simulink library "Kitchen_Lib"  (R2023a)
settings: Solver=VariableStepAuto  StartTime=0.0  StopTime=10.0  RelTol=1e-3  EnableMultiTasking=on
undefined symbols (not defined in the file): Kitc_BusTyp_P, Kitc_BusTypSkyr_C, Kitc_ColrLedColrls_C, Kitc_ColrLedGrn_C, Kitc_ColrLedRed_C, Kitc_ColrLedYlw_C, Kitc_StDgnWtrTank_C, Kitc_StElecPlugScktOffByClmp50_P, Kitc_StsDlyBlink_C, Kitc_StsErrBlink_C, Kitc_StsFctAcvn_P, Kitc_StsInfoBlink_C, Kitc_StsKitchnOffAutoIgOff_P, Kitc_StsKitchnOffBySwt_P, Kitc_StsKitchnOffDoorLockd_P, Kitc_StsKitchnOffIgOff_P, Kitc_StsKitchnOffUv_P, Kitc_StsKitchnOnBySwt_P, Kitc_StsKitchnOnNVM_P, Kitc_StsLedOff_C, Kitc_StsLedOn_C, Kitc_StsLrgCnsAcv_P, Kitc_StTrfrAnSwtInstd_P, Kitc_StTrfrSwtInstd_P, Kitc_TiKitcRefgtrOffDly_P, Kitc_ULowrThdBat_C, Kitc_UUpprThdBat_C, Kitc_ValFalse_C, Kitc_ValPwmFreq2_C, Kitc_ValPwmFreq_C, Kitc_ValTrue_C
libraries: MAN_Library x50, E2E_Lib x3
(part 8 of 13)

== system Kitchen_Lib/Kitchen/100ms/Kitchn/Subsystem1/Subsystem19/KSW_Battery/BatteryVoltageUnder23V/TurnOffDelay ==
  TurnOffDelayEnable : Inport
  TurnOffDelayThreshold : Inport  Port=2
  Constant1 : Constant  Value=uint32(100)  OutDataTypeStr=uint32
  Constant10 : Constant  Value=uint32(CycleTime)  OutDataTypeStr=uint32
  Constant11 : Constant  Value=uint32(1)  OutDataTypeStr=uint32
  Constant12 : Constant  Value=uint32(10)  OutDataTypeStr=uint32
  Constant13 : Constant  Value=uint32(100)  OutDataTypeStr=uint32
  Constant14 : Constant  Value=uint32(1000)  OutDataTypeStr=uint32
  Multiport Switch2 : MultiPortSwitch  Inputs=4  SaturateOnIntegerOverflow=off  InputSameDT=off
  Terminator : Terminator
  TurnOffDelayOriginal : Subsystem  AncestorBlock=MAN_Library/BasicLibrary/TurnOffDelayOriginal
  TurnOffDelayFlag : Outport
  TurnOffDelayExpiredTime : Outport  Port=2
  wires:
  TurnOffDelayOriginal/2(TurnOffDelayExpiredTime) -> TurnOffDelayExpiredTime/1
  TurnOffDelayOriginal/1(TurnOffDelayFlag) -> TurnOffDelayFlag/1
  TurnOffDelayThreshold/1 -> TurnOffDelayOriginal/2(TurnOffDelayThreshold)
  TurnOffDelayEnable/1 -> TurnOffDelayOriginal/1(TurnOffDelayEnable)
  Constant11/1 -> Multiport Switch2/2
  Constant12/1 -> Multiport Switch2/3
  Constant14/1 -> Multiport Switch2/5
  Constant13/1 -> Multiport Switch2/4
  Constant10/1 -> Multiport Switch2/1
  Multiport Switch2/1 -> Terminator/1
  Constant1/1 -> TurnOffDelayOriginal/3(CycleTime)

== system Kitchen_Lib/Kitchen/100ms/Kitchn/Subsystem1/Subsystem19/KitchenEnable/001_HostessSideButton/001_HostessSideTopButton ==
  note: Parameter G_78_PARA_Enable_KuecheBeif_S is deleted
  note: Parameter
      | G_78_PARA_Enable_KuecheBeif_S
      | is deleted
  Kitc_StKitcHostsSideSwtUpprPart : Inport
  SwtLock : Inport  Port=2
  "GW_ModeExbn " : Inport  Port=3
  "GW_StUvTopPrio " : Inport  Port=4
  Constant1 : Constant  Value=Kitc_ValFalse_C
  Logical Operator10 : Logic  Operator=NOT  Inputs=4  AllPortsSameDT=off  OutDataTypeStr=boolean
  Logical Operator11 : Logic  Operator=OR  Inputs=3  AllPortsSameDT=off  OutDataTypeStr=boolean
  Logical Operator12 : Logic  Operator=NOT  Inputs=4  AllPortsSameDT=off  OutDataTypeStr=boolean
  Logical Operator9 : Logic  Inputs=3  AllPortsSameDT=off  OutDataTypeStr=boolean
  RisingEdgeDetection : Subsystem  AncestorBlock=MAN_Library/RisingEdgeDetection
  HostessSideTopButtonErr : Outport
  wires:
  Logical Operator10/1 -> Logical Operator9/2
  Constant1/1 -> Logical Operator12/1
  RisingEdgeDetection/1(Q) -> Logical Operator9/3
  "GW_ModeExbn "/1 -> Logical Operator10/1
  Logical Operator12/1 -> Logical Operator11/1
  Logical Operator11/1 -> Logical Operator9/1
  SwtLock/1 -> Logical Operator11/2
  Logical Operator9/1 -> HostessSideTopButtonErr/1
  "GW_StUvTopPrio "/1 -> Logical Operator11/3
  Kitc_StKitcHostsSideSwtUpprPart/1 -> RisingEdgeDetection/1(CLK)

== system Kitchen_Lib/Kitchen/100ms/Kitchn/Subsystem1/Subsystem19/KitchenEnable/001_HostessSideButton/002_HostessSideBottomButton ==
  note: Parameter G_78_PARA_Enable_KuecheBeif_S is deleted
  note: Parameter G_78_PARA_Enable_KuecheBeif_S is deleted
  Kitchn_On : Inport
  "GW_ModeExbn " : Inport  Port=2
  Kitc_StKitcHostsSideSwtBotmPart : Inport  Port=3
  SwtLock : Inport  Port=4
  Constant1 : Constant  Value=Kitc_ValFalse_C
  Constant2 : Constant  Value=Kitc_ValFalse_C
  Logical Operator14 : Logic  Inputs=3  AllPortsSameDT=off  OutDataTypeStr=boolean
  Logical Operator15 : Logic  Operator=OR  AllPortsSameDT=off  OutDataTypeStr=boolean
  Logical Operator{16..17,29..30} (4 alike) : Logic  Operator=NOT  Inputs=4  AllPortsSameDT=off  OutDataTypeStr=boolean
  Logical Operator28 : Logic  Inputs=5  AllPortsSameDT=off  OutDataTypeStr=boolean
  RisingEdgeDetection : Subsystem  AncestorBlock=MAN_Library/RisingEdgeDetection
  HostessSideBottomButtonErr : Outport
  HostessSideBottomButton_OFF : Outport  Port=2
  wires:
  Logical Operator29/1 -> Logical Operator28/2
  Logical Operator16/1 -> Logical Operator14/2
  Constant2/1 -> Logical Operator17/1
  RisingEdgeDetection/1(Q) -> Logical Operator14/3, Logical Operator28/1
  Logical Operator28/1 -> HostessSideBottomButton_OFF/1
  SwtLock/1 -> Logical Operator15/2, Logical Operator30/1
  Logical Operator30/1 -> Logical Operator28/3
  Constant1/1 -> Logical Operator28/5
  "GW_ModeExbn "/1 -> Logical Operator16/1, Logical Operator29/1
  Logical Operator17/1 -> Logical Operator15/1
  Logical Operator14/1 -> HostessSideBottomButtonErr/1
  Kitc_StKitcHostsSideSwtBotmPart/1 -> RisingEdgeDetection/1(CLK)
  Logical Operator15/1 -> Logical Operator14/1
  Kitchn_On/1 -> Logical Operator28/4

== system Kitchen_Lib/Kitchen/100ms/Kitchn/Subsystem1/Subsystem19/KitchenEnable/KitchenOffAutomaticIgnitionOff/Constant4            ==
  Constant11 : Constant  Value=uint32(hours)  OutDataTypeStr=uint32
  Constant12 : Constant  Value=uint32(minutes)  OutDataTypeStr=uint32
  Constant13 : Constant  Value=uint32(miliseconds)  OutDataTypeStr=uint32
  Constant14 : Constant  Value=uint32(60)  OutDataTypeStr=uint32
  Constant15 : Constant  Value=uint32(1000)  OutDataTypeStr=uint32
  Constant16 : Constant  Value=uint32(seconds)  OutDataTypeStr=uint32
  Constant17 : Constant  Value=uint32(1000)  OutDataTypeStr=uint32
  Constant7 : Constant  Value=uint32(60)  OutDataTypeStr=uint32
  Constant8 : Constant  Value=uint32(60)  OutDataTypeStr=uint32
  Constant9 : Constant  Value=uint32(1000)  OutDataTypeStr=uint32
  Data Type Conversion{1..2,4..8,13..19} (14 alike) : DataTypeConversion  OutDataTypeStr=uint32  SaturateOnIntegerOverflow=off  RndMeth=Floor
  Product1 : Product  Inputs=4  OutDataTypeStr=uint32
  Product2 : Product  Inputs=3  OutDataTypeStr=uint32
  Product4 : Product  OutDataTypeStr=uint32
  Sum1 : Sum  Inputs=++++  AccumDataTypeStr=uint32
  time : Outport
  wires:
  Sum1/1 -> Data Type Conversion5/1  "time"
  Data Type Conversion5/1 -> time/1
  Constant7/1 -> Data Type Conversion13/1
  Data Type Conversion13/1 -> Product1/1
  Constant8/1 -> Data Type Conversion14/1
  Data Type Conversion14/1 -> Product1/2
  Constant9/1 -> Data Type Conversion15/1
  Data Type Conversion15/1 -> Product1/3
  Constant11/1 -> Data Type Conversion16/1
  Data Type Conversion16/1 -> Product1/4
  Constant12/1 -> Data Type Conversion2/1
  Constant14/1 -> Data Type Conversion17/1
  Data Type Conversion17/1 -> Product2/1
  Constant15/1 -> Data Type Conversion18/1
  Data Type Conversion18/1 -> Product2/2
  Constant17/1 -> Data Type Conversion19/1
  Data Type Conversion19/1 -> Product4/1
  Constant16/1 -> Data Type Conversion1/1
  Product1/1 -> Data Type Conversion4/1
  Product2/1 -> Data Type Conversion6/1
  Product4/1 -> Data Type Conversion7/1
  Data Type Conversion1/1 -> Product4/2
  Data Type Conversion2/1 -> Product2/3
  Constant13/1 -> Data Type Conversion8/1
  Data Type Conversion4/1 -> Sum1/1
  Data Type Conversion6/1 -> Sum1/2
  Data Type Conversion7/1 -> Sum1/3
  Data Type Conversion8/1 -> Sum1/4

== system Kitchen_Lib/Kitchen/100ms/Kitchn/Subsystem1/Subsystem19/KitchenEnable/KitchenOffAutomaticIgnitionOff/RisingEdgeDetection2 ==
  CLK : Inport
  Constant : Constant  Value=boolean(1)  OutDataTypeStr=boolean
  Data Type Conversion1 : DataTypeConversion  OutDataTypeStr=boolean  SaturateOnIntegerOverflow=off  RndMeth=Floor
  Logical Operator : Logic  AllPortsSameDT=off  OutDataTypeStr=boolean
  Relational Operator : RelationalOperator  Operator=~=  OutDataTypeStr=boolean  InputSameDT=off
  Relational Operator1 : RelationalOperator  Operator===  OutDataTypeStr=boolean  InputSameDT=off
  Unit Delay : UnitDelay  SampleTime=-1  HasFrameUpgradeWarning=on
  Q : Outport
  wires:
  CLK/1 -> Data Type Conversion1/1
  Unit Delay/1 -> Relational Operator/1
  Relational Operator/1 -> Logical Operator/1
  Relational Operator1/1 -> Logical Operator/2
  Logical Operator/1 -> Q/1
  Constant/1 -> Relational Operator1/2
  Data Type Conversion1/1 -> Unit Delay/1, Relational Operator/2, Relational Operator1/1

== system Kitchen_Lib/Kitchen/100ms/Kitchn/Subsystem1/Subsystem19/KitchenEnable/KitchenOffAutomaticIgnitionOff/TurnOnDelay ==
  TurnOnDelayEnable : Inport
  TurnOnDelayThreshold : Inport  Port=2
  Constant1 : Constant  Value=uint32(100)  OutDataTypeStr=uint32
  Constant11 : Constant  Value=uint32(1)  OutDataTypeStr=uint32
  Constant12 : Constant  Value=uint32(10)  OutDataTypeStr=uint32
  Constant13 : Constant  Value=uint32(100)  OutDataTypeStr=uint32
  Constant14 : Constant  Value=uint32(1000)  OutDataTypeStr=uint32
  Constant2 : Constant  Value=uint32(CycleTime)  OutDataTypeStr=uint32
  Multiport Switch2 : MultiPortSwitch  Inputs=4  SaturateOnIntegerOverflow=off  InputSameDT=off
  Terminator : Terminator
  TurnOnDelayOriginal : Subsystem  AncestorBlock=MAN_Library/BasicLibrary/TurnOnDelayOriginal
  TurnOnDelayFlag : Outport
  TurnOnDelayExpiredTime : Outport  Port=2
  wires:
  TurnOnDelayEnable/1 -> TurnOnDelayOriginal/1(TurnOnDelayEnable)
  TurnOnDelayThreshold/1 -> TurnOnDelayOriginal/2(TurnOnDelayThreshold)
  TurnOnDelayOriginal/2(TurnOnDelayExpiredTime) -> TurnOnDelayExpiredTime/1
  TurnOnDelayOriginal/1(TurnOnDelayFlag) -> TurnOnDelayFlag/1
  Constant11/1 -> Multiport Switch2/2
  Constant12/1 -> Multiport Switch2/3
  Constant14/1 -> Multiport Switch2/5
  Constant13/1 -> Multiport Switch2/4
  Constant2/1 -> Multiport Switch2/1
  Multiport Switch2/1 -> Terminator/1
  Constant1/1 -> TurnOnDelayOriginal/3(CycleTime)

== system Kitchen_Lib/Kitchen/100ms/Kitchn/Subsystem1/Subsystem19/KitchenEnable/KitchenOffDoorLocked/RisingEdgeDetection3 ==
  CLK : Inport
  Constant : Constant  Value=boolean(1)  OutDataTypeStr=boolean
  Data Type Conversion1 : DataTypeConversion  OutDataTypeStr=boolean  SaturateOnIntegerOverflow=off  RndMeth=Floor
  Logical Operator : Logic  AllPortsSameDT=off  OutDataTypeStr=boolean
  Relational Operator : RelationalOperator  Operator=~=  OutDataTypeStr=boolean  InputSameDT=off
  Relational Operator1 : RelationalOperator  Operator===  OutDataTypeStr=boolean  InputSameDT=off
  Unit Delay : UnitDelay  SampleTime=-1  HasFrameUpgradeWarning=on
  Q : Outport
  wires:
  CLK/1 -> Data Type Conversion1/1
  Unit Delay/1 -> Relational Operator/1
  Relational Operator/1 -> Logical Operator/1
  Relational Operator1/1 -> Logical Operator/2
  Logical Operator/1 -> Q/1
  Constant/1 -> Relational Operator1/2
  Data Type Conversion1/1 -> Unit Delay/1, Relational Operator/2, Relational Operator1/1

== system Kitchen_Lib/Kitchen/100ms/Kitchn/Subsystem1/Subsystem19/KitchenEnable/KitchenOffIgnitionOff/FallingEdgeDetection ==
  CLK : Inport
  Constant : Constant  Value=boolean(0)  OutDataTypeStr=boolean
  Data Type Conversion1 : DataTypeConversion  OutDataTypeStr=boolean  SaturateOnIntegerOverflow=off  RndMeth=Floor
  Logical Operator1 : Logic  AllPortsSameDT=off  OutDataTypeStr=boolean
  Relational Operator2 : RelationalOperator  Operator=~=  OutDataTypeStr=boolean  InputSameDT=off
  Relational Operator3 : RelationalOperator  Operator===  OutDataTypeStr=boolean  InputSameDT=off
  Unit Delay1 : UnitDelay  SampleTime=-1  HasFrameUpgradeWarning=on
  Q : Outport
  wires:
  Unit Delay1/1 -> Relational Operator2/1
  Relational Operator2/1 -> Logical Operator1/1
  Relational Operator3/1 -> Logical Operator1/2
  Logical Operator1/1 -> Q/1
  CLK/1 -> Data Type Conversion1/1
  Constant/1 -> Relational Operator3/2
  Data Type Conversion1/1 -> Relational Operator3/1, Relational Operator2/2, Unit Delay1/1

== system Kitchen_Lib/Kitchen/100ms/Kitchn/Subsystem1/Subsystem19/KitchenEnable/KitchenOffUndervoltage/RisingEdgeDetection4 ==
  CLK : Inport
  Constant : Constant  Value=boolean(1)  OutDataTypeStr=boolean
  Data Type Conversion1 : DataTypeConversion  OutDataTypeStr=boolean  SaturateOnIntegerOverflow=off  RndMeth=Floor
  Logical Operator : Logic  AllPortsSameDT=off  OutDataTypeStr=boolean
  Relational Operator : RelationalOperator  Operator=~=  OutDataTypeStr=boolean  InputSameDT=off
  Relational Operator1 : RelationalOperator  Operator===  OutDataTypeStr=boolean  InputSameDT=off
  Unit Delay : UnitDelay  SampleTime=-1  HasFrameUpgradeWarning=on
  Q : Outport
  wires:
  CLK/1 -> Data Type Conversion1/1
  Unit Delay/1 -> Relational Operator/1
  Relational Operator/1 -> Logical Operator/1
  Relational Operator1/1 -> Logical Operator/2
  Logical Operator/1 -> Q/1
  Constant/1 -> Relational Operator1/2
  Data Type Conversion1/1 -> Unit Delay/1, Relational Operator/2, Relational Operator1/1

== system Kitchen_Lib/Kitchen/100ms/Kitchn/Subsystem1/Subsystem19/KitchenEnable/KitchenOnNVM/NVM ==
  KitchnOffBySwt : Inport
  HostsSideBotmBtn_OFF : Inport  Port=2
  "GW_StStrtNew " : Inport  Port=3
  Kitc_ModeKitcNv : Inport  Port=4
  Kitchn_On : Inport  Port=5
  GW_StClmp15 : Inport  Port=6
  Data Store Write : DataStoreWrite  DataStoreName=Kitc_ModeKitcNv  IndexOptions=Index vector (dialog)  Indices=1  OutputSizes=1
  Logical Operator41 : Logic  Operator=OR  Inputs=3  AllPortsSameDT=off  OutDataTypeStr=boolean
  Logical Operator{42..43,46,48} (4 alike) : Logic  AllPortsSameDT=off  OutDataTypeStr=boolean
  Logical Operator44 : Logic  Inputs=4  AllPortsSameDT=off  OutDataTypeStr=boolean
  Logical Operator45 : Logic  Operator=NOT  Inputs=4  AllPortsSameDT=off  OutDataTypeStr=boolean
  Logical Operator47 : Logic  Operator=NOT  Inputs=4  AllPortsSameDT=off  OutDataTypeStr=boolean
  Logical Operator49 : Logic  Operator=NOT  Inputs=4  AllPortsSameDT=off  OutDataTypeStr=boolean
  RisingEdgeDetection1 : Subsystem  AncestorBlock=MAN_Library/RisingEdgeDetection
  RisingEdgeDetection2 : Subsystem  AncestorBlock=MAN_Library/RisingEdgeDetection
  wires:
  Logical Operator48/1 -> Logical Operator49/1
  RisingEdgeDetection1/1(Q) -> Logical Operator42/1
  Logical Operator49/1 -> Logical Operator44/4
  Logical Operator44/1 -> Data Store Write/1
  Kitchn_On/1 -> Logical Operator42/2, RisingEdgeDetection2/1(CLK)
  Logical Operator45/1 -> Logical Operator44/2
  Logical Operator41/1 -> Logical Operator44/1
  Kitc_ModeKitcNv/1 -> Logical Operator41/1
  RisingEdgeDetection2/1(Q) -> Logical Operator43/1
  Logical Operator46/1 -> Logical Operator47/1
  Logical Operator43/1 -> Logical Operator41/3
  Logical Operator42/1 -> Logical Operator41/2
  Logical Operator47/1 -> Logical Operator44/3
  GW_StClmp15/1 -> RisingEdgeDetection1/1(CLK), Logical Operator48/1, Logical Operator46/1, Logical Operator43/2
  KitchnOffBySwt/1 -> Logical Operator46/2
  HostsSideBotmBtn_OFF/1 -> Logical Operator48/2
  "GW_StStrtNew "/1 -> Logical Operator45/1

== system Kitchen_Lib/Kitchen/100ms/Kitchn/Subsystem1/Subsystem19/KitchenEnable/KitchenOnNVM/NvM_ActiveOnlyForFirstCycle ==
  NVM_Bool_In : Inport
  Constant2 : Constant  Value=boolean(1)  OutDataTypeStr=boolean
  Constant3 : Constant  Value=boolean(0)  OutDataTypeStr=boolean
  Data Type Conversion2 : DataTypeConversion  OutDataTypeStr=boolean  SaturateOnIntegerOverflow=off  RndMeth=Floor
  Logical Operator : Logic  AllPortsSameDT=off  OutDataTypeStr=boolean
  Unit Delay External IC : Subsystem  AncestorBlock=|  mask(Unit Delay External Initial Condition){tsamp=-1}
      | simulink/Additional Math
      | & Discrete/Additional
      | Discrete/Unit Delay
      | External IC
      mask prompts: tsamp "Simulink:masks:SampleTime_MP"
      mask help: Simulink:masks:UnitDelayExternalInitialCondition_MD
      mask Display: dpoly(1,[1 0],'z')
  NVM_Bool_Out : Outport
  wires:
  NVM_Bool_In/1 -> Data Type Conversion2/1
  Logical Operator/1 -> NVM_Bool_Out/1
  Unit Delay External IC/1(y) -> Logical Operator/2
  Constant3/1 -> Unit Delay External IC/1(u)
  Constant2/1 -> Unit Delay External IC/2(IC)
  Data Type Conversion2/1 -> Logical Operator/1

== system Kitchen_Lib/Kitchen/100ms/Kitchn/Subsystem1/Subsystem19/KitchenEnable/KitchenOnNVM/RisingEdgeDetection5 ==
  CLK : Inport
  Constant : Constant  Value=boolean(1)  OutDataTypeStr=boolean
  Data Type Conversion1 : DataTypeConversion  OutDataTypeStr=boolean  SaturateOnIntegerOverflow=off  RndMeth=Floor
  Logical Operator : Logic  AllPortsSameDT=off  OutDataTypeStr=boolean
  Relational Operator : RelationalOperator  Operator=~=  OutDataTypeStr=boolean  InputSameDT=off
  Relational Operator1 : RelationalOperator  Operator===  OutDataTypeStr=boolean  InputSameDT=off
  Unit Delay : UnitDelay  SampleTime=-1  HasFrameUpgradeWarning=on
  Q : Outport
  wires:
  CLK/1 -> Data Type Conversion1/1
  Unit Delay/1 -> Relational Operator/1
  Relational Operator/1 -> Logical Operator/1
  Relational Operator1/1 -> Logical Operator/2
  Logical Operator/1 -> Q/1
  Constant/1 -> Relational Operator1/2
  Data Type Conversion1/1 -> Unit Delay/1, Relational Operator/2, Relational Operator1/1

== system Kitchen_Lib/Kitchen/100ms/Kitchn/Subsystem1/Subsystem19/KitchenEnable/Subsystem/RS ==
  S : Inport
  R : Inport  Port=2
  Constant2 : Constant  Value=boolean(1)  OutDataTypeStr=boolean
  Constant3 : Constant  Value=boolean(0)  OutDataTypeStr=boolean
  Data Type Conversion1 : DataTypeConversion  OutDataTypeStr=boolean  SaturateOnIntegerOverflow=off  RndMeth=Floor
  Data Type Conversion2 : DataTypeConversion  OutDataTypeStr=boolean  SaturateOnIntegerOverflow=off  RndMeth=Floor
  Multiport Switch : MultiPortSwitch  DataPortOrder=Zero-based contiguous  Inputs=2  zeroidx=on  SaturateOnIntegerOverflow=off  InputSameDT=off
  Multiport Switch2 : MultiPortSwitch  DataPortOrder=Zero-based contiguous  Inputs=2  zeroidx=on  SaturateOnIntegerOverflow=off  InputSameDT=off
  Unit Delay : UnitDelay  SampleTime=-1  HasFrameUpgradeWarning=on
  Q : Outport
  wires:
  Data Type Conversion1/1 -> Multiport Switch2/1
  Data Type Conversion2/1 -> Multiport Switch/1
  Multiport Switch2/1 -> Unit Delay/1, Q/1
  Multiport Switch/1 -> Multiport Switch2/2
  Constant3/1 -> Multiport Switch2/3
  R/1 -> Data Type Conversion1/1
  Unit Delay/1 -> Multiport Switch/2
  Constant2/1 -> Multiport Switch/3
  S/1 -> Data Type Conversion2/1

== system Kitchen_Lib/Kitchen/100ms/Kitchn/Subsystem1/Subsystem19/KitchenEnable/Subsystem/RisingEdgeDetection ==
  CLK : Inport
  Constant : Constant  Value=boolean(1)  OutDataTypeStr=boolean
  Data Type Conversion1 : DataTypeConversion  OutDataTypeStr=boolean  SaturateOnIntegerOverflow=off  RndMeth=Floor
  Logical Operator : Logic  AllPortsSameDT=off  OutDataTypeStr=boolean
  Relational Operator : RelationalOperator  Operator=~=  OutDataTypeStr=boolean  InputSameDT=off
  Relational Operator1 : RelationalOperator  Operator===  OutDataTypeStr=boolean  InputSameDT=off
  Unit Delay : UnitDelay  SampleTime=-1  HasFrameUpgradeWarning=on
  Q : Outport
  wires:
  Data Type Conversion1/1 -> Relational Operator1/1, Relational Operator/2, Unit Delay/1
  Constant/1 -> Relational Operator1/2
  Logical Operator/1 -> Q/1
  Relational Operator1/1 -> Logical Operator/2
  Relational Operator/1 -> Logical Operator/1
  Unit Delay/1 -> Relational Operator/1
  CLK/1 -> Data Type Conversion1/1

== system Kitchen_Lib/Kitchen/100ms/Kitchn/Subsystem1/Subsystem19/KitchenEnable/Subsystem/StateChangePulse ==
  note: This function replaces '2k+1 XOR' block to detect changes.
  IN : Inport
  Data Type Conversion1 : DataTypeConversion  OutDataTypeStr=boolean  SaturateOnIntegerOverflow=off  RndMeth=Floor
  Data Type Conversion2 : DataTypeConversion  Commented=on  OutDataTypeStr=boolean  SaturateOnIntegerOverflow=off  RndMeth=Floor
  Ground : Ground  Commented=on
  Logical Operator17 : Logic  Operator=XOR  AllPortsSameDT=off  OutDataTypeStr=boolean
  Relational Operator : RelationalOperator  Commented=on  Operator=~=  OutDataTypeStr=boolean  InputSameDT=off
  Terminator : Terminator  Commented=on
  Unit Delay : UnitDelay  SampleTime=-1  HasFrameUpgradeWarning=on
  Unit Delay1 : UnitDelay  Commented=on  SampleTime=-1  HasFrameUpgradeWarning=on
  OUT : Outport
  wires:
  Unit Delay1/1 -> Relational Operator/1
  IN/1 -> Data Type Conversion1/1
  Ground/1 -> Data Type Conversion2/1
  Relational Operator/1 -> Terminator/1
  Data Type Conversion2/1 -> Unit Delay1/1, Relational Operator/2
  Data Type Conversion1/1 -> Logical Operator17/1
  Unit Delay/1 -> Logical Operator17/2
  Logical Operator17/1 -> Unit Delay/1, OUT/1

== system Kitchen_Lib/Kitchen/100ms/Kitchn/Subsystem1/Subsystem19/KitchenEnable/Subsystem/TimeConstant ==
  Constant11 : Constant  Value=uint32(hours)  OutDataTypeStr=uint32
  Constant12 : Constant  Value=uint32(minutes)  OutDataTypeStr=uint32
  Constant13 : Constant  Value=uint32(miliseconds)  OutDataTypeStr=uint32
  Constant14 : Constant  Value=uint32(60)  OutDataTypeStr=uint32
  Constant15 : Constant  Value=uint32(1000)  OutDataTypeStr=uint32
  Constant16 : Constant  Value=uint32(seconds)  OutDataTypeStr=uint32
  Constant17 : Constant  Value=uint32(1000)  OutDataTypeStr=uint32
  Constant7 : Constant  Value=uint32(60)  OutDataTypeStr=uint32
  Constant8 : Constant  Value=uint32(60)  OutDataTypeStr=uint32
  Constant9 : Constant  Value=uint32(1000)  OutDataTypeStr=uint32
  Data Type Conversion{1..2,4..8,13..19} (14 alike) : DataTypeConversion  OutDataTypeStr=uint32  SaturateOnIntegerOverflow=off  RndMeth=Floor
  Product1 : Product  Inputs=4  OutDataTypeStr=uint32
  Product2 : Product  Inputs=3  OutDataTypeStr=uint32
  Product4 : Product  OutDataTypeStr=uint32
  Sum1 : Sum  Inputs=++++  AccumDataTypeStr=uint32
  time : Outport
  wires:
  Data Type Conversion8/1 -> Sum1/4
  Data Type Conversion7/1 -> Sum1/3
  Data Type Conversion6/1 -> Sum1/2
  Data Type Conversion4/1 -> Sum1/1
  Constant13/1 -> Data Type Conversion8/1
  Data Type Conversion2/1 -> Product2/3
  Data Type Conversion1/1 -> Product4/2
  Product4/1 -> Data Type Conversion7/1
  Product2/1 -> Data Type Conversion6/1
  Product1/1 -> Data Type Conversion4/1
  Constant16/1 -> Data Type Conversion1/1
  Data Type Conversion19/1 -> Product4/1
  Constant17/1 -> Data Type Conversion19/1
  Data Type Conversion18/1 -> Product2/2
  Constant15/1 -> Data Type Conversion18/1
  Data Type Conversion17/1 -> Product2/1
  Constant14/1 -> Data Type Conversion17/1
  Constant12/1 -> Data Type Conversion2/1
  Data Type Conversion16/1 -> Product1/4
  Constant11/1 -> Data Type Conversion16/1
  Data Type Conversion15/1 -> Product1/3
  Constant9/1 -> Data Type Conversion15/1
  Data Type Conversion14/1 -> Product1/2
  Constant8/1 -> Data Type Conversion14/1
  Data Type Conversion13/1 -> Product1/1
  Constant7/1 -> Data Type Conversion13/1
  Data Type Conversion5/1 -> time/1
  Sum1/1 -> Data Type Conversion5/1  "time"

== system Kitchen_Lib/Kitchen/100ms/Kitchn/Subsystem1/Subsystem19/KitchenEnable/Subsystem/TurnOnDelay ==
  TurnOnDelayEnable : Inport
  TurnOnDelayThreshold : Inport  Port=2
  Constant10 : Constant  Value=uint32(CycleTime)  OutDataTypeStr=uint32
  Constant16 : Constant  Value=uint32(1)  OutDataTypeStr=uint32
  Constant17 : Constant  Value=uint32(10)  OutDataTypeStr=uint32
  Constant18 : Constant  Value=uint32(100)  OutDataTypeStr=uint32
  Constant19 : Constant  Value=uint32(1000)  OutDataTypeStr=uint32
  Multiport Switch4 : MultiPortSwitch  Inputs=4  SaturateOnIntegerOverflow=off  InputSameDT=off
  TurnOnDelayOriginal : Subsystem  AncestorBlock=MAN_Library/BasicLibrary/TurnOnDelayOriginal
  TurnOnDelayFlag : Outport
  TurnOnDelayExpiredTime : Outport  Port=2
  wires:
  TurnOnDelayOriginal/1(TurnOnDelayFlag) -> TurnOnDelayFlag/1
  TurnOnDelayOriginal/2(TurnOnDelayExpiredTime) -> TurnOnDelayExpiredTime/1
  TurnOnDelayThreshold/1 -> TurnOnDelayOriginal/2(TurnOnDelayThreshold)
  TurnOnDelayEnable/1 -> TurnOnDelayOriginal/1(TurnOnDelayEnable)
  Constant19/1 -> Multiport Switch4/5
  Constant18/1 -> Multiport Switch4/4
  Constant17/1 -> Multiport Switch4/3
  Constant16/1 -> Multiport Switch4/2
  Constant10/1 -> Multiport Switch4/1
  Multiport Switch4/1 -> TurnOnDelayOriginal/3(CycleTime)

== system Kitchen_Lib/Kitchen/100ms/Kitchn/Subsystem1/Subsystem19/KitchenSwtLed/KitchenError/RisingEdgeDetection ==
  CLK : Inport
  Constant : Constant  Value=boolean(1)  OutDataTypeStr=boolean
  Data Type Conversion1 : DataTypeConversion  OutDataTypeStr=boolean  SaturateOnIntegerOverflow=off  RndMeth=Floor
  Logical Operator : Logic  AllPortsSameDT=off  OutDataTypeStr=boolean
  Relational Operator : RelationalOperator  Operator=~=  OutDataTypeStr=boolean  InputSameDT=off
  Relational Operator1 : RelationalOperator  Operator===  OutDataTypeStr=boolean  InputSameDT=off
  Unit Delay : UnitDelay  SampleTime=-1  HasFrameUpgradeWarning=on
  Q : Outport
  wires:
  CLK/1 -> Data Type Conversion1/1
  Unit Delay/1 -> Relational Operator/1
  Relational Operator/1 -> Logical Operator/1
  Relational Operator1/1 -> Logical Operator/2
  Logical Operator/1 -> Q/1
  Constant/1 -> Relational Operator1/2
  Data Type Conversion1/1 -> Unit Delay/1, Relational Operator/2, Relational Operator1/1

== system Kitchen_Lib/Kitchen/100ms/Kitchn/Subsystem1/Subsystem19/KitchenSwtLed/KitchenError/TurnOffDelay ==
  TurnOffDelayEnable : Inport
  TurnOffDelayThreshold : Inport  Port=2
  Constant1 : Constant  Value=uint32(100)  OutDataTypeStr=uint32
  Constant10 : Constant  Value=uint32(CycleTime)  OutDataTypeStr=uint32
  Constant11 : Constant  Value=uint32(1)  OutDataTypeStr=uint32
  Constant12 : Constant  Value=uint32(10)  OutDataTypeStr=uint32
  Constant13 : Constant  Value=uint32(100)  OutDataTypeStr=uint32
  Constant14 : Constant  Value=uint32(1000)  OutDataTypeStr=uint32
  Multiport Switch2 : MultiPortSwitch  Inputs=4  SaturateOnIntegerOverflow=off  InputSameDT=off
  Terminator : Terminator
  TurnOffDelayOriginal : Subsystem  AncestorBlock=MAN_Library/BasicLibrary/TurnOffDelayOriginal
  TurnOffDelayFlag : Outport
  TurnOffDelayExpiredTime : Outport  Port=2
  wires:
  TurnOffDelayOriginal/2(TurnOffDelayExpiredTime) -> TurnOffDelayExpiredTime/1
  TurnOffDelayOriginal/1(TurnOffDelayFlag) -> TurnOffDelayFlag/1
  TurnOffDelayThreshold/1 -> TurnOffDelayOriginal/2(TurnOffDelayThreshold)
  TurnOffDelayEnable/1 -> TurnOffDelayOriginal/1(TurnOffDelayEnable)
  Constant11/1 -> Multiport Switch2/2
  Constant12/1 -> Multiport Switch2/3
  Constant14/1 -> Multiport Switch2/5
  Constant13/1 -> Multiport Switch2/4
  Constant10/1 -> Multiport Switch2/1
  Multiport Switch2/1 -> Terminator/1
  Constant1/1 -> TurnOffDelayOriginal/3(CycleTime)

== system Kitchen_Lib/Kitchen/100ms/Kitchn/Subsystem1/Subsystem19/KitchenSwtLed/TurnOffDelay1/TurnOffDelayOriginal ==
  TurnOffDelayEnable : Inport
  TurnOffDelayThreshold : Inport  Port=2
  CycleTime : Inport  Port=3
  Data Type Conversion1 : DataTypeConversion  OutDataTypeStr=uint32  SaturateOnIntegerOverflow=off  RndMeth=Floor
  Data Type Conversion2 : DataTypeConversion  OutDataTypeStr=boolean  SaturateOnIntegerOverflow=off  RndMeth=Floor
  Data Type Conversion3 : DataTypeConversion  OutDataTypeStr=uint32  SaturateOnIntegerOverflow=off  RndMeth=Floor
  FallingEdgeDetection : Subsystem  AncestorBlock=MAN_Library/FallingEdgeDetection
  Logical Operator2 : Logic  Operator=OR  AllPortsSameDT=off  OutDataTypeStr=boolean
  TimePulseOriginal : Subsystem  AncestorBlock=MAN_Library/BasicLibrary/TimePulseOriginal
  TurnOffDelayFlag : Outport
  TurnOffDelayExpiredTime : Outport  Port=2
  wires:
  CycleTime/1 -> TimePulseOriginal/3(CycleTime)
  Data Type Conversion3/1 -> TurnOffDelayExpiredTime/1
  Data Type Conversion1/1 -> TimePulseOriginal/2(TimePulseDuration)
  TurnOffDelayThreshold/1 -> Data Type Conversion1/1
  FallingEdgeDetection/1(Q) -> TimePulseOriginal/1(TimePulseEnable)
  TimePulseOriginal/2(TimePulseExpiredTime) -> Data Type Conversion3/1
  Logical Operator2/1 -> TurnOffDelayFlag/1
  TimePulseOriginal/1(TimePulseFlag) -> Logical Operator2/2
  Data Type Conversion2/1 -> FallingEdgeDetection/1(CLK), Logical Operator2/1
  TurnOffDelayEnable/1 -> Data Type Conversion2/1

== system Kitchen_Lib/Kitchen/100ms/Kitchn/Subsystem1/Subsystem19/Refgtr/TurnOffDelay/TurnOffDelayOriginal ==
  TurnOffDelayEnable : Inport
  TurnOffDelayThreshold : Inport  Port=2
  CycleTime : Inport  Port=3
  Data Type Conversion1 : DataTypeConversion  OutDataTypeStr=uint32  SaturateOnIntegerOverflow=off  RndMeth=Floor
  Data Type Conversion2 : DataTypeConversion  OutDataTypeStr=boolean  SaturateOnIntegerOverflow=off  RndMeth=Floor
  Data Type Conversion3 : DataTypeConversion  OutDataTypeStr=uint32  SaturateOnIntegerOverflow=off  RndMeth=Floor
  FallingEdgeDetection : Subsystem  AncestorBlock=MAN_Library/FallingEdgeDetection
  Logical Operator2 : Logic  Operator=OR  AllPortsSameDT=off  OutDataTypeStr=boolean
  TimePulseOriginal : Subsystem  AncestorBlock=MAN_Library/BasicLibrary/TimePulseOriginal
  TurnOffDelayFlag : Outport
  TurnOffDelayExpiredTime : Outport  Port=2
  wires:
  CycleTime/1 -> TimePulseOriginal/3(CycleTime)
  Data Type Conversion3/1 -> TurnOffDelayExpiredTime/1
  Data Type Conversion1/1 -> TimePulseOriginal/2(TimePulseDuration)
  TurnOffDelayThreshold/1 -> Data Type Conversion1/1
  FallingEdgeDetection/1(Q) -> TimePulseOriginal/1(TimePulseEnable)
  TimePulseOriginal/2(TimePulseExpiredTime) -> Data Type Conversion3/1
  Logical Operator2/1 -> TurnOffDelayFlag/1
  TimePulseOriginal/1(TimePulseFlag) -> Logical Operator2/2
  Data Type Conversion2/1 -> FallingEdgeDetection/1(CLK), Logical Operator2/1
  TurnOffDelayEnable/1 -> Data Type Conversion2/1

== system Kitchen_Lib/Kitchen/100ms/Kitchn/Subsystem1/Subsystem19/TimePulse/TimePulseOriginal/RisingEdgeDetection ==
  CLK : Inport
  Constant : Constant  Value=boolean(1)  OutDataTypeStr=boolean
  Data Type Conversion1 : DataTypeConversion  OutDataTypeStr=boolean  SaturateOnIntegerOverflow=off  RndMeth=Floor
  Logical Operator : Logic  AllPortsSameDT=off  OutDataTypeStr=boolean
  Relational Operator : RelationalOperator  Operator=~=  OutDataTypeStr=boolean  InputSameDT=off
  Relational Operator1 : RelationalOperator  Operator===  OutDataTypeStr=boolean  InputSameDT=off
  Unit Delay : UnitDelay  SampleTime=-1  HasFrameUpgradeWarning=on
  Q : Outport
  wires:
  Data Type Conversion1/1 -> Relational Operator1/1, Relational Operator/2, Unit Delay/1
  Constant/1 -> Relational Operator1/2
  Logical Operator/1 -> Q/1
  Relational Operator1/1 -> Logical Operator/2
  Relational Operator/1 -> Logical Operator/1
  Unit Delay/1 -> Relational Operator/1
  CLK/1 -> Data Type Conversion1/1

== system Kitchen_Lib/Kitchen/100ms/Kitchn/Subsystem1/Subsystem19/TimePulse/TimePulseOriginal/RisingEdgeDetection1 ==
  CLK : Inport
  Constant : Constant  Value=boolean(1)  OutDataTypeStr=boolean
  Data Type Conversion1 : DataTypeConversion  OutDataTypeStr=boolean  SaturateOnIntegerOverflow=off  RndMeth=Floor
  Logical Operator : Logic  AllPortsSameDT=off  OutDataTypeStr=boolean
  Relational Operator : RelationalOperator  Operator=~=  OutDataTypeStr=boolean  InputSameDT=off
  Relational Operator1 : RelationalOperator  Operator===  OutDataTypeStr=boolean  InputSameDT=off
  Unit Delay : UnitDelay  SampleTime=-1  HasFrameUpgradeWarning=on
  Q : Outport
  wires:
  Data Type Conversion1/1 -> Relational Operator1/1, Relational Operator/2, Unit Delay/1
  Constant/1 -> Relational Operator1/2
  Logical Operator/1 -> Q/1
  Relational Operator1/1 -> Logical Operator/2
  Relational Operator/1 -> Logical Operator/1
  Unit Delay/1 -> Relational Operator/1
  CLK/1 -> Data Type Conversion1/1

== system Kitchen_Lib/Kitchen/100ms/Kitchn/Subsystem1/Subsystem19/TimePulse/TimePulseOriginal/SR ==
  S : Inport
  R : Inport  Port=2
  Constant1 : Constant  Value=boolean(1)  OutDataTypeStr=boolean
  Constant3 : Constant  Value=boolean(0)  OutDataTypeStr=boolean
  Data Type Conversion1 : DataTypeConversion  OutDataTypeStr=boolean  SaturateOnIntegerOverflow=off  RndMeth=Floor
  Data Type Conversion2 : DataTypeConversion  OutDataTypeStr=boolean  SaturateOnIntegerOverflow=off  RndMeth=Floor
  Multiport Switch : MultiPortSwitch  DataPortOrder=Zero-based contiguous  Inputs=2  zeroidx=on  SaturateOnIntegerOverflow=off  InputSameDT=off
  Multiport Switch1 : MultiPortSwitch  DataPortOrder=Zero-based contiguous  Inputs=2  zeroidx=on  SaturateOnIntegerOverflow=off  InputSameDT=off
  Unit Delay : UnitDelay  SampleTime=-1  HasFrameUpgradeWarning=on
  Q : Outport
  wires:
  Data Type Conversion2/1 -> Multiport Switch/1
  Data Type Conversion1/1 -> Multiport Switch1/1
  Constant3/1 -> Multiport Switch1/3
  Multiport Switch/1 -> Unit Delay/1, Q/1
  Unit Delay/1 -> Multiport Switch1/2
  R/1 -> Data Type Conversion1/1
  Multiport Switch1/1 -> Multiport Switch/2
  Constant1/1 -> Multiport Switch/3
  S/1 -> Data Type Conversion2/1

== system Kitchen_Lib/Kitchen/100ms/Kitchn/Subsystem1/Subsystem19/TimePulse/TimePulseOriginal/TimerCountingUpOriginal ==
  TimerEnable : Inport
  TimerReset : Inport  Port=2
  TimerThreshold : Inport  Port=3
  CycleTime : Inport  Port=4
  Data Type Conversion2 : DataTypeConversion  OutDataTypeStr=boolean  SaturateOnIntegerOverflow=off  RndMeth=Floor
  Data Type Conversion4 : DataTypeConversion  OutDataTypeStr=uint32  SaturateOnIntegerOverflow=off  RndMeth=Floor
  Data Type Conversion5 : DataTypeConversion  OutDataTypeStr=uint32  SaturateOnIntegerOverflow=off  RndMeth=Floor
  Data Type Conversion6 : DataTypeConversion  OutDataTypeStr=uint32  SaturateOnIntegerOverflow=off  RndMeth=Floor
  Data Type Conversion7 : DataTypeConversion  OutDataTypeStr=boolean  SaturateOnIntegerOverflow=off  RndMeth=Floor
  Delay : Delay  DelayLength=1  InitialCondition=0  ExternalReset=Rising
      settings: InputPortMap=u0,r5
  Delay1 : Delay  DelayLength=1  InitialCondition=0
  Logical Operator1 : Logic  Operator=NOT  AllPortsSameDT=off  OutDataTypeStr=boolean
  Logical Operator2 : Logic  AllPortsSameDT=off  OutDataTypeStr=boolean
  Logical Operator3 : Logic  Operator=OR  AllPortsSameDT=off  OutDataTypeStr=boolean
  Multiport Switch : MultiPortSwitch  DataPortOrder=Zero-based contiguous  Inputs=2  zeroidx=on  SaturateOnIntegerOverflow=off  InputSameDT=off
  Multiport Switch1 : MultiPortSwitch  DataPortOrder=Zero-based contiguous  Inputs=2  zeroidx=on  SaturateOnIntegerOverflow=off  InputSameDT=off
  Multiport Switch2 : MultiPortSwitch  DataPortOrder=Zero-based contiguous  Inputs=2  zeroidx=on  SaturateOnIntegerOverflow=off  InputSameDT=off
  Relational Operator : RelationalOperator  OutDataTypeStr=boolean  InputSameDT=off
  Relational Operator1 : RelationalOperator  Operator===  OutDataTypeStr=boolean  InputSameDT=off
  RisingEdgeDetection : Subsystem  AncestorBlock=MAN_Library/RisingEdgeDetection
  StartValue_ms1 : Constant  Value=uint32(4294967295)  OutDataTypeStr=uint32
  StartValue_ms2 : Constant  Value=uint32(4294967295)  OutDataTypeStr=uint32
  StartValue_ms3 : Constant  Value=uint32(0)  OutDataTypeStr=uint32
  StartValue_ms5 : Constant  Value=uint32(4294967295)  OutDataTypeStr=uint32
  Sum : Sum
  U32_Saturation : Subsystem  AncestorBlock=MAN_Library/U32_Saturation
  TimerFlag : Outport
  TimerCurrentValue : Outport  Port=2
  wires:
  CycleTime/1 -> Data Type Conversion4/1
  Data Type Conversion2/1 -> Logical Operator3/1
  RisingEdgeDetection/1(Q) -> Logical Operator3/2
  TimerReset/1 -> Data Type Conversion2/1
  TimerEnable/1 -> Data Type Conversion7/1
  Data Type Conversion6/1 -> Relational Operator/2
  Data Type Conversion4/1 -> Sum/2
  StartValue_ms3/1 -> U32_Saturation/3(LowerLimit), Multiport Switch/3
  Multiport Switch2/1 -> U32_Saturation/2(IN)
  Sum/1 -> Multiport Switch2/2
  StartValue_ms2/1 -> Multiport Switch2/3
  Relational Operator1/1 -> Multiport Switch2/1
  Delay/1 -> Multiport Switch1/2, Relational Operator1/1, Sum/1
  StartValue_ms5/1 -> Relational Operator1/2
  Logical Operator3/1 -> Multiport Switch/1, [ResetTimer_BOOL]
  StartValue_ms1/1 -> U32_Saturation/1(UpperLimit)
  Delay1/1 -> Logical Operator1/1
  U32_Saturation/1(OUT) -> Multiport Switch1/3
  Logical Operator1/1 -> Logical Operator2/2
  Logical Operator2/1 -> Multiport Switch1/1
  Data Type Conversion5/1 -> TimerCurrentValue/1, Delay/1, Relational Operator/1
  Data Type Conversion7/1 -> Logical Operator2/1, RisingEdgeDetection/1(CLK)
  Multiport Switch/1 -> Data Type Conversion5/1
  Relational Operator/1 -> TimerFlag/1, Delay1/1
  Multiport Switch1/1 -> Multiport Switch/2
  TimerThreshold/1 -> Data Type Conversion6/1
  [ResetTimer_BOOL] -> Delay/2

== system Kitchen_Lib/Kitchen/100ms/Kitchn/Subsystem1/Subsystem19/Trfr/002_FlipFlop/KSW-Nvm ==
  TurnOn : Inport
  TurnOff : Inport  Port=2
  "GW_StStrtNew " : Inport  Port=3
  Kitc_StTrfrWoutNewStrt : Inport  Port=4
  Data Store Write : DataStoreWrite  DataStoreName=Kitc_StsTurnOnByBtnNv  IndexOptions=Index vector (dialog)  Indices=1  OutputSizes=1
  Logical Operator : Logic  Operator=OR  AllPortsSameDT=off  OutDataTypeStr=boolean
  Logical Operator1 : Logic  Operator=NOT  AllPortsSameDT=off  OutDataTypeStr=boolean
  Logical Operator2 : Logic  AllPortsSameDT=off  OutDataTypeStr=boolean
  SR : Subsystem  AncestorBlock=MAN_Library/SR
  wires:
  TurnOn/1 -> SR/1(S)
  Logical Operator/1 -> SR/2(R)
  Kitc_StTrfrWoutNewStrt/1 -> Logical Operator1/1
  Logical Operator1/1 -> Logical Operator2/2
  "GW_StStrtNew "/1 -> Logical Operator2/1
  Logical Operator2/1 -> Logical Operator/2
  TurnOff/1 -> Logical Operator/1
  SR/1(Q) -> Data Store Write/1

== system Kitchen_Lib/Kitchen/100ms/Kitchn/Subsystem1/Subsystem19/Trfr/002_FlipFlop/NvM_ActiveOnlyForFirstCycle ==
  NVM_Bool_In : Inport
  Constant2 : Constant  Value=boolean(1)  OutDataTypeStr=boolean
  Constant3 : Constant  Value=boolean(0)  OutDataTypeStr=boolean
  Data Type Conversion2 : DataTypeConversion  OutDataTypeStr=boolean  SaturateOnIntegerOverflow=off  RndMeth=Floor
  Logical Operator : Logic  AllPortsSameDT=off  OutDataTypeStr=boolean
  Unit Delay External IC : Subsystem  AncestorBlock=|  mask(Unit Delay External Initial Condition){tsamp=-1}
      | simulink/Additional Math
      | & Discrete/Additional
      | Discrete/Unit Delay
      | External IC
      mask prompts: tsamp "Simulink:masks:SampleTime_MP"
      mask help: Simulink:masks:UnitDelayExternalInitialCondition_MD
      mask Display: dpoly(1,[1 0],'z')
  NVM_Bool_Out : Outport
  wires:
  NVM_Bool_In/1 -> Data Type Conversion2/1
  Logical Operator/1 -> NVM_Bool_Out/1
  Unit Delay External IC/1(y) -> Logical Operator/2
  Constant3/1 -> Unit Delay External IC/1(u)
  Constant2/1 -> Unit Delay External IC/2(IC)
  Data Type Conversion2/1 -> Logical Operator/1

== system Kitchen_Lib/Kitchen/100ms/Kitchn/Subsystem1/Subsystem19/Trfr/002_FlipFlop/StateChangePulse ==
  note: This function replaces '2k+1 XOR' block to detect changes.
  IN : Inport
  Data Type Conversion1 : DataTypeConversion  OutDataTypeStr=boolean  SaturateOnIntegerOverflow=off  RndMeth=Floor
  Data Type Conversion2 : DataTypeConversion  Commented=on  OutDataTypeStr=boolean  SaturateOnIntegerOverflow=off  RndMeth=Floor
  Ground : Ground  Commented=on
  Logical Operator17 : Logic  Operator=XOR  AllPortsSameDT=off  OutDataTypeStr=boolean
  Relational Operator : RelationalOperator  Commented=on  Operator=~=  OutDataTypeStr=boolean  InputSameDT=off
  Terminator : Terminator  Commented=on
  Unit Delay : UnitDelay  SampleTime=-1  HasFrameUpgradeWarning=on
  Unit Delay1 : UnitDelay  Commented=on  SampleTime=-1  HasFrameUpgradeWarning=on
  OUT : Outport
  wires:
  Logical Operator17/1 -> OUT/1, Unit Delay/1
  Unit Delay/1 -> Logical Operator17/2
  Data Type Conversion1/1 -> Logical Operator17/1
  Data Type Conversion2/1 -> Relational Operator/2, Unit Delay1/1
  Relational Operator/1 -> Terminator/1
  Ground/1 -> Data Type Conversion2/1
  IN/1 -> Data Type Conversion1/1
  Unit Delay1/1 -> Relational Operator/1

== system Kitchen_Lib/Kitchen/100ms/Kitchn/Subsystem1/Subsystem19/Trfr/002_FlipFlop/TurnOffByButton ==
  Kitc_StTrfrSwtLowrPart : Inport
  Kitc_StTrfrBotmBtm : Inport  Port=2
  Fnc_ON : Inport  Port=3
  Logical Operator11 : Logic  AllPortsSameDT=off  OutDataTypeStr=boolean
  Logical Operator9 : Logic  Operator=OR  AllPortsSameDT=off  OutDataTypeStr=boolean
  RisingEdgeDetection1 : Subsystem  AncestorBlock=MAN_Library/RisingEdgeDetection
  TurnOff : Outport
  wires:
  Kitc_StTrfrBotmBtm/1 -> Logical Operator9/2
  RisingEdgeDetection1/1(Q) -> Logical Operator11/1
  Logical Operator9/1 -> RisingEdgeDetection1/1(CLK)
  Fnc_ON/1 -> Logical Operator11/2
  Kitc_StTrfrSwtLowrPart/1 -> Logical Operator9/1
  Logical Operator11/1 -> TurnOff/1

== system Kitchen_Lib/Kitchen/100ms/Kitchn/Subsystem1/Subsystem19/Trfr/002_FlipFlop/TurnOffConditions ==
  GW_StEngRung : Inport
  ABat_StAddlBatInstd : Inport  Port=2
  GW_StClmp15 : Inport  Port=3
  "GW_StUvNormPrio " : Inport  Port=4
  Fnc_ON : Inport  Port=5
  FallingEdgeDetection : Subsystem  AncestorBlock=MAN_Library/FallingEdgeDetection
  FallingEdgeDetection1 : Subsystem  AncestorBlock=MAN_Library/FallingEdgeDetection
  Logical Operator13 : Logic  AllPortsSameDT=off  OutDataTypeStr=boolean
  Logical Operator14 : Logic  Operator=NOT  AllPortsSameDT=off  OutDataTypeStr=boolean
  Logical Operator15 : Logic  Operator=OR  Inputs=3  AllPortsSameDT=off  OutDataTypeStr=boolean
  Logical Operator16 : Logic  AllPortsSameDT=off  OutDataTypeStr=boolean
  RisingEdgeDetection2 : Subsystem  AncestorBlock=MAN_Library/RisingEdgeDetection
  CdnOff : Outport
  wires:
  "GW_StUvNormPrio "/1 -> RisingEdgeDetection2/1(CLK)
  Logical Operator14/1 -> Logical Operator16/2
  RisingEdgeDetection2/1(Q) -> Logical Operator15/2
  GW_StEngRung/1 -> FallingEdgeDetection1/1(CLK)
  Logical Operator15/1 -> Logical Operator13/2
  FallingEdgeDetection/1(Q) -> Logical Operator15/1
  Fnc_ON/1 -> Logical Operator13/1
  FallingEdgeDetection1/1(Q) -> Logical Operator16/1
  ABat_StAddlBatInstd/1 -> Logical Operator14/1
  Logical Operator16/1 -> Logical Operator15/3
  Logical Operator13/1 -> CdnOff/1
  GW_StClmp15/1 -> FallingEdgeDetection/1(CLK)

== system Kitchen_Lib/Kitchen/100ms/Kitchn/Subsystem1/Subsystem19/Trfr/002_FlipFlop/TurnOnByButton ==
  Kitc_StTrfrSwtUpprPart : Inport
  Kitc_StTrfrSwtTopBtn : Inport  Port=2
  GW_StEngRung : Inport  Port=3
  ABat_StAddlBatInstd : Inport  Port=4
  GW_StClmp15 : Inport  Port=5
  "GW_StUvNormPrio " : Inport  Port=6
  Fnc_ON : Inport  Port=7
  Logical Operator10 : Logic  Operator=NOT  AllPortsSameDT=off  OutDataTypeStr=boolean
  Logical Operator12 : Logic  Operator=OR  AllPortsSameDT=off  OutDataTypeStr=boolean
  Logical Operator6 : Logic  Inputs=5  AllPortsSameDT=off  OutDataTypeStr=boolean
  Logical Operator7 : Logic  Operator=NOT  AllPortsSameDT=off  OutDataTypeStr=boolean
  Logical Operator8 : Logic  Operator=OR  AllPortsSameDT=off  OutDataTypeStr=boolean
  RisingEdgeDetection : Subsystem  AncestorBlock=MAN_Library/RisingEdgeDetection
  TurnOn : Outport
  wires:
  RisingEdgeDetection/1(Q) -> Logical Operator6/5
  Logical Operator10/1 -> Logical Operator6/3
  Logical Operator12/1 -> Logical Operator6/1
  Fnc_ON/1 -> Logical Operator7/1
  Kitc_StTrfrSwtUpprPart/1 -> Logical Operator8/1
  ABat_StAddlBatInstd/1 -> Logical Operator12/2
  "GW_StUvNormPrio "/1 -> Logical Operator10/1
  Logical Operator7/1 -> Logical Operator6/4
  Kitc_StTrfrSwtTopBtn/1 -> Logical Operator8/2
  GW_StClmp15/1 -> Logical Operator6/2
  GW_StEngRung/1 -> Logical Operator12/1
  Logical Operator8/1 -> RisingEdgeDetection/1(CLK)
  Logical Operator6/1 -> TurnOn/1

== system Kitchen_Lib/Kitchen/100ms/Kitchn/Subsystem1/Subsystem19/Trfr/002_FlipFlop/TurnOnNvm ==
  TrfrSwt : Inport
  Kitc_StsTurnOnByBtnNv : Inport  Port=2
  GW_StEngRung : Inport  Port=3
  ABat_StAddlBatInstd : Inport  Port=4
  GW_StClmp15 : Inport  Port=5
  Fnc_ON : Inport  Port=6
  GW_StUvNormPrio : Inport  Port=7
  Kitc_StsTurnOnByBtnNv1 : DataStoreWrite  DataStoreName=Kitc_StsTurnOnByBtnNv  IndexOptions=Index vector (dialog)  Indices=1  OutputSizes=1
  Logical Operator17 : Logic  Inputs=5  AllPortsSameDT=off  OutDataTypeStr=boolean
  Logical Operator18 : Logic  Operator=NOT  AllPortsSameDT=off  OutDataTypeStr=boolean
  Logical Operator19 : Logic  Operator=NOT  AllPortsSameDT=off  OutDataTypeStr=boolean
  Logical Operator20 : Logic  AllPortsSameDT=off  OutDataTypeStr=boolean
  Logical Operator21 : Logic  Operator=OR  AllPortsSameDT=off  OutDataTypeStr=boolean
  RisingEdgeDetection3 : Subsystem  AncestorBlock=MAN_Library/RisingEdgeDetection
  RisingEdgeDetection4 : Subsystem  AncestorBlock=MAN_Library/RisingEdgeDetection
  TurnOnNvm : Outport
  wires:
  Kitc_StsTurnOnByBtnNv/1 -> Logical Operator17/4
  Logical Operator20/1 -> Logical Operator21/2
  Fnc_ON/1 -> Logical Operator18/1
  RisingEdgeDetection3/1(Q) -> Logical Operator21/1
  ABat_StAddlBatInstd/1 -> Logical Operator20/2
  Logical Operator19/1 -> Logical Operator17/3
  GW_StUvNormPrio/1 -> Logical Operator19/1
  Logical Operator18/1 -> Logical Operator17/2
  RisingEdgeDetection4/1(Q) -> Logical Operator20/1
  Logical Operator21/1 -> Logical Operator17/5
  GW_StClmp15/1 -> RisingEdgeDetection4/1(CLK)
  TrfrSwt/1 -> Logical Operator17/1
  Logical Operator17/1 -> Kitc_StsTurnOnByBtnNv1/1, TurnOnNvm/1
  GW_StEngRung/1 -> RisingEdgeDetection3/1(CLK)

== system Kitchen_Lib/Kitchen/100ms/Kitchn/Subsystem1/Subsystem19/Trfr/TurnOnDelay/TurnOnDelayOriginal ==
  TurnOnDelayEnable : Inport
  TurnOnDelayThreshold : Inport  Port=2
  CycleTime : Inport  Port=3
  Data Type Conversion1 : DataTypeConversion  OutDataTypeStr=uint32  SaturateOnIntegerOverflow=off  RndMeth=Floor
  Data Type Conversion2 : DataTypeConversion  OutDataTypeStr=boolean  SaturateOnIntegerOverflow=off  RndMeth=Floor
  Logical Operator1 : Logic  Operator=NOT  AllPortsSameDT=off  OutDataTypeStr=boolean
  Logical Operator2 : Logic  AllPortsSameDT=off  OutDataTypeStr=boolean
  RisingEdgeDetection : Subsystem  AncestorBlock=MAN_Library/RisingEdgeDetection
  TimePulseOriginal : Subsystem  AncestorBlock=MAN_Library/BasicLibrary/TimePulseOriginal
  TurnOnDelayFlag : Outport
  TurnOnDelayExpiredTime : Outport  Port=2
  wires:
  CycleTime/1 -> TimePulseOriginal/3(CycleTime)
  Logical Operator2/1 -> TurnOnDelayFlag/1
  TimePulseOriginal/1(TimePulseFlag) -> Logical Operator1/1
  Logical Operator1/1 -> Logical Operator2/2
  TimePulseOriginal/2(TimePulseExpiredTime) -> TurnOnDelayExpiredTime/1
  RisingEdgeDetection/1(Q) -> TimePulseOriginal/1(TimePulseEnable)
  Data Type Conversion1/1 -> TimePulseOriginal/2(TimePulseDuration)
  TurnOnDelayThreshold/1 -> Data Type Conversion1/1
  TurnOnDelayEnable/1 -> Data Type Conversion2/1
  Data Type Conversion2/1 -> RisingEdgeDetection/1(CLK), Logical Operator2/1

== system Kitchen_Lib/Kitchen/100ms/Kitchn/Subsystem1/Subsystem19/WaterTankEmptyDiagnostic/Diagno sticsDebouncing/DiagnosticsDebouncingOriginal ==
  Error : Inport
  StartLock : Inport  Port=2
  IgnitionStatus : Inport  Port=3
  OnDelay : Inport  Port=4
  OffDelay : Inport  Port=5
  CycleTime : Inport  Port=6
  Data Type Conversion1 : DataTypeConversion  OutDataTypeStr=boolean  SaturateOnIntegerOverflow=off  RndMeth=Floor
  Data Type Conversion2 : DataTypeConversion  OutDataTypeStr=boolean  SaturateOnIntegerOverflow=off  RndMeth=Floor
  Data Type Conversion3 : DataTypeConversion  OutDataTypeStr=boolean  SaturateOnIntegerOverflow=off  RndMeth=Floor
  Data Type Conversion4 : DataTypeConversion  OutDataTypeStr=uint32  SaturateOnIntegerOverflow=off  RndMeth=Floor
  Data Type Conversion5 : DataTypeConversion  OutDataTypeStr=uint32  SaturateOnIntegerOverflow=off  RndMeth=Floor
  Logical Operator : Logic  Operator=NOT  Inputs=1  AllPortsSameDT=off  OutDataTypeStr=boolean
  Logical Operator1 : Logic  Inputs=4  AllPortsSameDT=off  OutDataTypeStr=boolean
  Logical Operator2 : Logic  AllPortsSameDT=off  OutDataTypeStr=boolean
  Logical Operator3 : Logic  AllPortsSameDT=off  OutDataTypeStr=boolean
  Logical Operator4 : Logic  Operator=NOT  Inputs=1  AllPortsSameDT=off  OutDataTypeStr=boolean
  RS : Subsystem  AncestorBlock=MAN_Library/RS
  Terminator : Terminator
  Terminator1 : Terminator
  "TurnOffDelayOriginal " : Subsystem  AncestorBlock=MAN_Library/BasicLibrary/TurnOffDelayOriginal
  TurnOnDelayOriginal : Subsystem  AncestorBlock=MAN_Library/BasicLibrary/TurnOnDelayOriginal
  DiagnosticFlag : Outport
  wires:
  Data Type Conversion5/1 -> "TurnOffDelayOriginal "/2(TurnOffDelayThreshold)
  CycleTime/1 -> TurnOnDelayOriginal/3(CycleTime), "TurnOffDelayOriginal "/3(CycleTime)
  RS/1(Q) -> DiagnosticFlag/1
  [ViewError] -> Logical Operator4/1
  Logical Operator4/1 -> RS/2(R)
  Logical Operator1/1 -> RS/1(S)
  [IgnitionStatus] -> Logical Operator1/4
  Logical Operator2/1 -> [ViewError], Logical Operator1/3
  "TurnOffDelayOriginal "/1(TurnOffDelayFlag) -> Logical Operator2/2
  [IgnitionStatus] -> Logical Operator2/1
  Data Type Conversion1/1 -> Logical Operator3/1, Logical Operator1/1
  Logical Operator/1 -> Logical Operator1/2
  Data Type Conversion2/1 -> Logical Operator/1
  "TurnOffDelayOriginal "/2(TurnOffDelayExpiredTime) -> Terminator1/1
  TurnOnDelayOriginal/2(TurnOnDelayExpiredTime) -> Terminator/1
  TurnOnDelayOriginal/1(TurnOnDelayFlag) -> "TurnOffDelayOriginal "/1(TurnOffDelayEnable)
  Data Type Conversion4/1 -> TurnOnDelayOriginal/2(TurnOnDelayThreshold)
  Logical Operator3/1 -> TurnOnDelayOriginal/1(TurnOnDelayEnable)
  Data Type Conversion3/1 -> Logical Operator3/2, [IgnitionStatus]
  Error/1 -> Data Type Conversion1/1
  StartLock/1 -> Data Type Conversion2/1
  IgnitionStatus/1 -> Data Type Conversion3/1
  OnDelay/1 -> Data Type Conversion4/1
  OffDelay/1 -> Data Type Conversion5/1
